simulink model "rezervoar_poredjenje"  (R2016a)
settings: Solver=FixedStepAuto  StartTime=0.0  StopTime=1000.0  FixedStep=0.01  RelTol=1e-3
values from neighbouring files (symbols this model uses):
  A = -A0/A1 * (g / sqrt(2*g*h0))    [postavljanje_konstanti.m]
  A0 = 0.01    [postavljanje_konstanti.m]
  A1 = 2    [postavljanje_konstanti.m]
  B = 1/A1    (= 0.5)    [postavljanje_konstanti.m]
  C = 1    [postavljanje_konstanti.m]
  D = 0    [postavljanje_konstanti.m]
  g = 9.81    [postavljanje_konstanti.m]
  h0 = 5    [postavljanje_konstanti.m]
  q0 = A0 * sqrt(2*g*h0)    [postavljanje_konstanti.m]
  qu_max = 0.099    [postavljanje_konstanti.m]
settings Model: Creator=Vukan  LastModifiedBy=Vukan

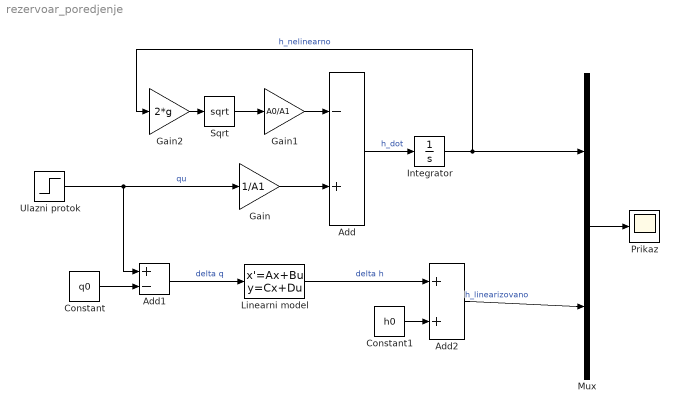
== system rezervoar_poredjenje ==
  Add : Sum  Inputs=-+
  Add1 : Sum  Inputs=+-
  Add2 : Sum
  Constant : Constant  Value=q0
  Constant1 : Constant  Value=h0
  Gain : Gain  Gain=1/A1
  Gain1 : Gain  Gain=A0/A1
  Gain2 : Gain  Gain=2*g
  Integrator : Integrator
  Linearni model : StateSpace  A=A  B=B  C=C  D=D  X0=0
  Mux : Mux  Inputs=2
  Prikaz : Scope
  Sqrt : Sqrt  SaturateOnIntegerOverflow=on
  Ulazni protok : Step  Time=100  After=qu_max  SampleTime=0
  wires:
  Gain/1 -> Add/2
  Add/1 -> Integrator/1  "h_dot"
  Integrator/1 -> Gain2/1, Mux/1  "h_nelinearno"
  Sqrt/1 -> Gain1/1
  Gain2/1 -> Sqrt/1
  Gain1/1 -> Add/1
  Constant/1 -> Add1/2
  Add1/1 -> Linearni model/1  "delta q"
  Linearni model/1 -> Add2/1  "delta h"
  Constant1/1 -> Add2/2
  Mux/1 -> Prikaz/1
  Add2/1 -> Mux/2  "h_linearizovano"
  Ulazni protok/1 -> Add1/1, Gain/1  "qu"
